simulink subsystem "airframe_propulsion"  (R2023b)
settings: Solver=VariableStepAuto  StartTime=0.0  StopTime=10.0  RelTol=1e-3
undefined symbols (not defined in the file): C_Q, C_T, D, i_0, K_Q, K_V, p, R_motor, V_max
settings Model: Creator=Victor  LastModifiedBy=Victor

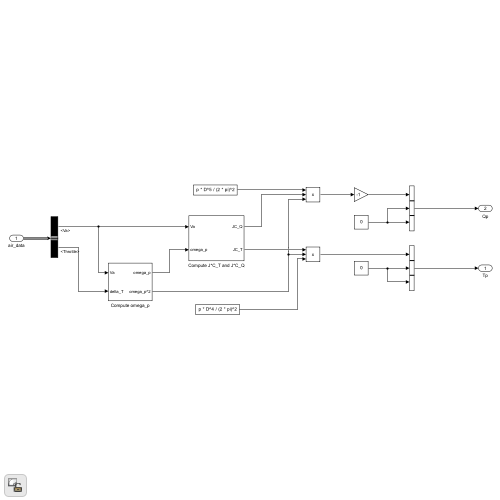
[thumbnail: Simulink's stored preview of the top-level diagram]
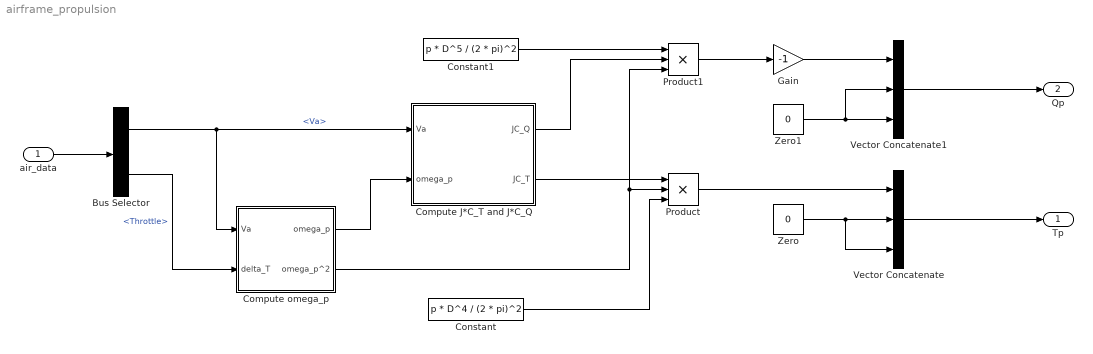
== system airframe_propulsion ==
  air_data : Inport
  Bus Selector : BusSelector  OutputSignals=target.Va,control.Throttle
  Compute J*C_T and J*C_Q : Subsystem
  Compute omega_p : Subsystem
  Constant : Constant  Value=p * D^4 / (2 * pi)^2
  Constant1 : Constant  Value=p * D^5 / (2 * pi)^2
  Gain : Gain  Gain=-1
  Product : Product  Inputs=3
  Product1 : Product  Inputs=3
  Vector Concatenate : Concatenate  NumInputs=3
  Vector Concatenate1 : Concatenate  NumInputs=3
  Zero : Constant  Value=0  OutDataTypeStr=Inherit: Inherit via back propagation
  Zero1 : Constant  Value=0  OutDataTypeStr=Inherit: Inherit via back propagation
  Tp : Outport
  Qp : Outport  Port=2
  wires:
  Constant/1 -> Product/3
  Compute J*C_T and J*C_Q/1(JC_Q) -> Product1/2
  Bus Selector/2 -> Compute omega_p/2(delta_T)  "<Throttle>"
  Constant1/1 -> Product1/1
  Compute J*C_T and J*C_Q/2(JC_T) -> Product/1
  Bus Selector/1 -> Compute J*C_T and J*C_Q/1(Va), Compute omega_p/1(Va)  "<Va>"
  Compute omega_p/1(omega_p) -> Compute J*C_T and J*C_Q/2(omega_p)
  Compute omega_p/2(omega_p^2) -> Product/2, Product1/3
  Product1/1 -> Gain/1
  Product/1 -> Vector Concatenate/1
  air_data/1 -> Bus Selector/1
  Gain/1 -> Vector Concatenate1/1
  Vector Concatenate1/1 -> Qp/1
  Zero1/1 -> Vector Concatenate1/2, Vector Concatenate1/3
  Vector Concatenate/1 -> Tp/1
  Zero/1 -> Vector Concatenate/2, Vector Concatenate/3

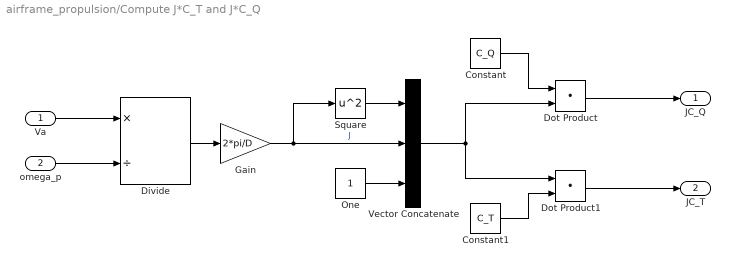
== system airframe_propulsion/Compute J*C_T and J*C_Q ==
  Va : Inport
  omega_p : Inport  Port=2
  Constant : Constant  Value=C_Q
  Constant1 : Constant  Value=C_T
  Divide : Product  Inputs=*/
  Dot Product : DotProduct  OutDataTypeStr=Inherit: Inherit via internal rule
  Dot Product1 : DotProduct  OutDataTypeStr=Inherit: Inherit via internal rule
  Gain : Gain  Gain=2*pi/D
  One : Constant  OutDataTypeStr=Inherit: Inherit via back propagation
  Square : Math  Operator=square
  Vector Concatenate : Concatenate  NumInputs=3
  JC_Q : Outport
  JC_T : Outport  Port=2
  wires:
  Va/1 -> Divide/1
  omega_p/1 -> Divide/2
  Divide/1 -> Gain/1
  Gain/1 -> Square/1, Vector Concatenate/2  "J"
  Square/1 -> Vector Concatenate/1
  One/1 -> Vector Concatenate/3
  Constant/1 -> Dot Product/1
  Vector Concatenate/1 -> Dot Product1/1, Dot Product/2
  Constant1/1 -> Dot Product1/2
  Dot Product1/1 -> JC_T/1
  Dot Product/1 -> JC_Q/1

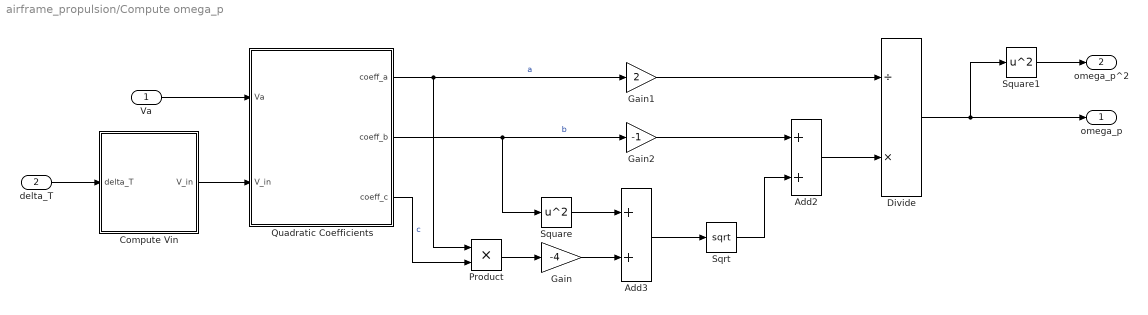
== system airframe_propulsion/Compute omega_p ==
  Va : Inport
  delta_T : Inport  Port=2
  Add2 : Sum
  Add3 : Sum
  Compute Vin : Subsystem
  Divide : Product  Inputs=/*
  Gain : Gain  Gain=-4
  Gain1 : Gain  Gain=2
  Gain2 : Gain  Gain=-1
  Product : Product
  Quadratic Coefficients : Subsystem
  Sqrt : Sqrt
  Square : Math  Operator=square
  Square1 : Math  Operator=square
  omega_p : Outport
  omega_p^2 : Outport  Port=2
  wires:
  delta_T/1 -> Compute Vin/1(delta_T)
  Product/1 -> Gain/1
  Divide/1 -> omega_p/1, Square1/1
  Va/1 -> Quadratic Coefficients/1(Va)
  Compute Vin/1(V_in) -> Quadratic Coefficients/2(V_in)
  Square1/1 -> omega_p^2/1
  Quadratic Coefficients/1(coeff_a) -> Product/1, Gain1/1  "a"
  Gain1/1 -> Divide/1
  Quadratic Coefficients/2(coeff_b) -> Square/1, Gain2/1  "b"
  Gain2/1 -> Add2/1
  Sqrt/1 -> Add2/2
  Add3/1 -> Sqrt/1
  Square/1 -> Add3/1
  Gain/1 -> Add3/2
  Quadratic Coefficients/3(coeff_c) -> Product/2  "c"
  Add2/1 -> Divide/2

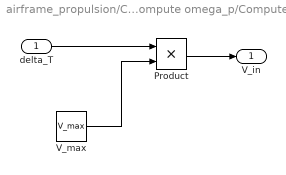
== system airframe_propulsion/Compute omega_p/Compute Vin ==
  delta_T : Inport
  Product : Product
  V_max : Constant  Value=V_max
  V_in : Outport
  wires:
  V_max/1 -> Product/2
  Product/1 -> V_in/1
  delta_T/1 -> Product/1

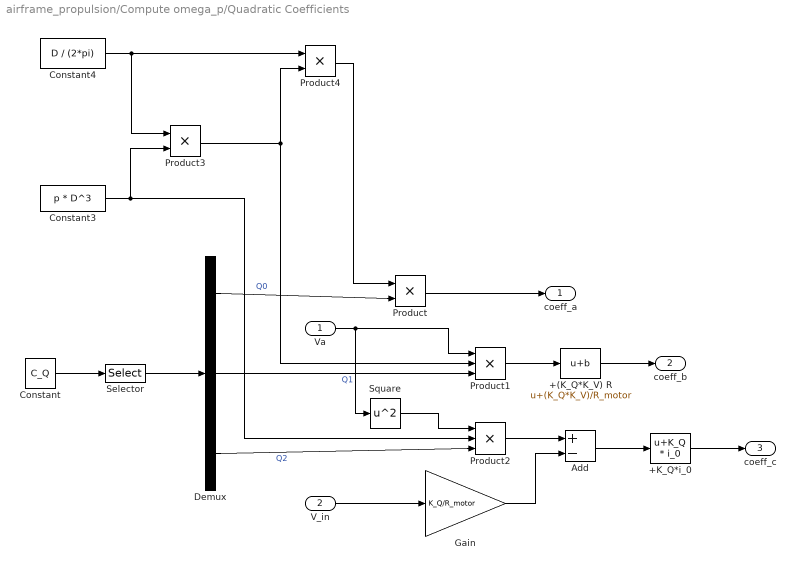
== system airframe_propulsion/Compute omega_p/Quadratic Coefficients ==
  Va : Inport
  V_in : Inport  Port=2
  +(K_Q*K_V) R : Bias  Bias=(K_Q*K_V)/R_motor  SaturateOnIntegerOverflow=off
  +K_Q*i_0 : Bias  Bias=K_Q * i_0  SaturateOnIntegerOverflow=off
  Add : Sum  Inputs=+-
  Constant : Constant  Value=C_Q
  Constant3 : Constant  Value=p * D^3
  Constant4 : Constant  Value=D / (2*pi)
  Demux : Demux  Outputs=3
  Gain : Gain  Gain=K_Q/R_motor
  Product : Product
  Product1 : Product  Inputs=3
  Product2 : Product  Inputs=3
  Product3 : Product
  Product4 : Product
  Selector : Selector  InputPortWidth=3  IndexOptions=Index vector (dialog)  Indices=[3 2 1]  OutputSizes=1
  Square : Math  Operator=square
  coeff_a : Outport
  coeff_b : Outport  Port=2
  coeff_c : Outport  Port=3
  wires:
  Constant3/1 -> Product2/2, Product3/2
  Constant4/1 -> Product4/1, Product3/1
  Product3/1 -> Product1/2, Product4/2
  Constant/1 -> Selector/1
  Selector/1 -> Demux/1
  Demux/1 -> Product/2  "Q0"
  Demux/2 -> Product1/3  "Q1"
  Demux/3 -> Product2/3  "Q2"
  Product4/1 -> Product/1
  Product/1 -> coeff_a/1
  Va/1 -> Square/1, Product1/1
  Product1/1 -> +(K_Q*K_V) R/1
  +(K_Q*K_V) R/1 -> coeff_b/1
  Square/1 -> Product2/1
  Product2/1 -> Add/1
  V_in/1 -> Gain/1
  Gain/1 -> Add/2
  Add/1 -> +K_Q*i_0/1
  +K_Q*i_0/1 -> coeff_c/1
